simulink model "five"  (R2020b)
settings: Solver=VariableStepAuto  StartTime=0.0  StopTime=10.0  RelTol=1e-3
undefined symbols (not defined in the file): C, R
settings Model: Creator=Dell  LastModifiedBy=Dell

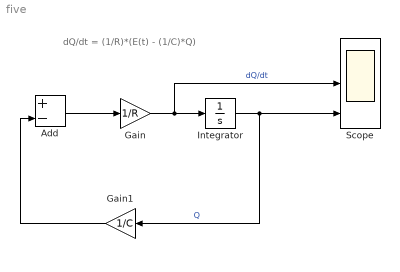
== system five ==
  note: dQ/dt = (1/R)*(E(t) - (1/C)*Q)
  Add : Sum  Inputs=+-
  Gain : Gain  Gain=1/R
  Gain1 : Gain  Gain=1/C
  Integrator : Integrator
  Scope : Scope  NumInputPorts=3
  wires:
  Add/1 -> Gain/1
  Gain/1 -> Scope/2, Integrator/1  "dQ/dt"
  Integrator/1 -> Gain1/1, Scope/3  "Q"
  Gain1/1 -> Add/2
  ? -> Scope/1, Add/1  "E(t)"
